simulink model "VVI"  (R2022b)
settings: Solver=FixedStepAuto  StartTime=0.0  StopTime=10.0  FixedStep=1e-3  RelTol=1e-3  EnableMultiTasking=on
undefined symbols (not defined in the file): D1, D10, D11, D12, D13, D2, D3, D4, D5, D7, D8, D9, PTA0, PTA1, PTA2, PTB23, PTB9, PTC17, PTC3, PTC4, PTD0, PTD1, PTD2, PTD3
libraries: frdmk64flib x12
settings Model: ExtModeTrigDuration=5  Creator=16475  LastModifiedBy=16475
settings OptimizationCC: EnhancedBackFolding=on  PassReuseOutputArgsAs=Individual arguments  ZeroExternalMemoryAtStartup=off  ZeroInternalMemoryAtStartup=off  MaxStackSize=64  OptimizeBlockOrder=speed  DifferentSizesBufferReuse=on  OptimizationCustomize=off  EfficientTunableParamExpr=on
settings DebuggingCC: ParameterTunabilityLossMsg=error
settings HardwareCC: ProdBitPerPointer=32  ProdBitPerSizeT=32  ProdBitPerPtrDiffT=32  ProdLargestAtomicInteger=Long  ProdLargestAtomicFloat=Double  ProdWordSize=32  ProdHWDeviceType=ARM Compatible->ARM Cortex
settings SFSimCC: MATLABDynamicMemAlloc=off
settings RTWCC: Description=Embedded Coder  SystemTargetFile=ert.tlc  HardwareBoard=NXP FRDM-K64F  TLCOptions="-aInlineSetEventsForThisBaseRateFcn=TLC_FALSE -aSuppressMultiTaskScheduler=TLC_FALSE  -aRateBasedStepFcn=0"  TemplateMakefile=ert_default_tmf  Toolchain=GNU Tools for ARM Embedded Processors
settings CodeAppCC: ForceParamTrailComments=on  IgnoreCustomStorageClasses=off  OperatorAnnotations=on  SimulinkDataObjDesc=on  SFDataObjDesc=on  InsertBlockDesc=on
settings ERTTargetCC: ExtModeTransport=4  ExtModeMexFile=sendToCommService

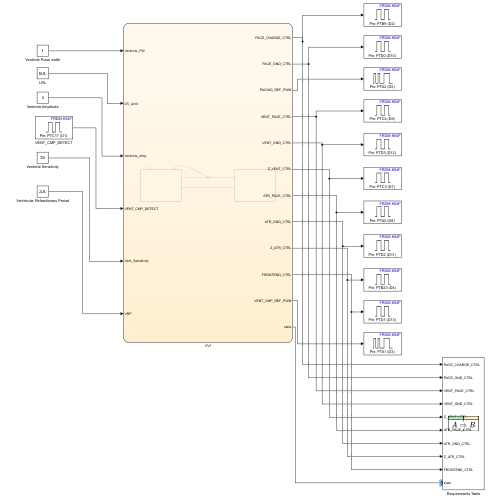
[thumbnail: Simulink's stored preview of the top-level diagram]
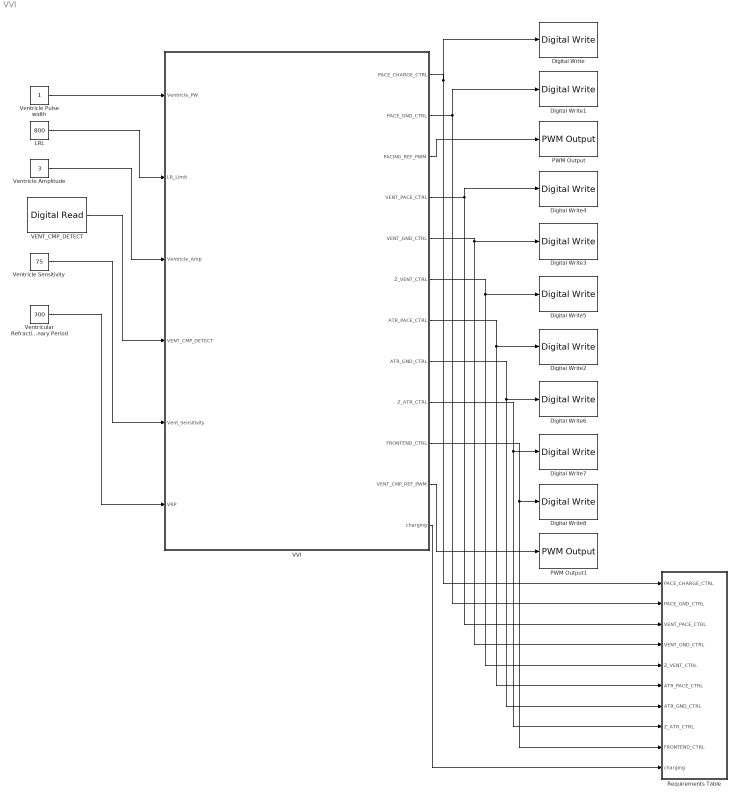
== system VVI ==
  Digital Write : frdmk64flib/Digital Write  Whichpin=PTB9 (D2)
  Digital Write1 : frdmk64flib/Digital Write  Whichpin=PTD0 (D10)
  Digital Write2 : frdmk64flib/Digital Write  Whichpin=PTA0 (D8)
  Digital Write3 : frdmk64flib/Digital Write  Whichpin=PTD3 (D12)
  Digital Write4 : frdmk64flib/Digital Write  Whichpin=PTC4 (D9)
  Digital Write5 : frdmk64flib/Digital Write  Whichpin=PTC3 (D7)
  Digital Write6 : frdmk64flib/Digital Write  Whichpin=PTD2 (D11)
  Digital Write7 : frdmk64flib/Digital Write  Whichpin=PTB23 (D4)
  Digital Write8 : frdmk64flib/Digital Write  Whichpin=PTD1 (D13)
  LRL : Constant  Value=800
  PWM Output : frdmk64flib/PWM Output  Whichpin=PTA2 (D5)  InitialFrequency=2000  InitialDutyCycle=0
  PWM Output1 : frdmk64flib/PWM Output  Whichpin=PTA1 (D3)  InitialFrequency=2000  InitialDutyCycle=0
  Requirements Table : Requirements Table  TreatAsAtomicUnit=on
  VENT_CMP_DETECT : frdmk64flib/Digital Read  Whichpin=PTC17 (D1)  SampleTime=-1
  VVI : Stateflow chart  TreatAsAtomicUnit=on
      settings: PortSchema="{\"entries\":[{\"content\":{\"sides\":[{\"content\":{\"connectorIds\":[\"In1\",\"In2\",\"In3\",\"In4\",\"In5\",\"In6\"]},\"type\":\"ConnectorPlacement.EquallySpacedRectSide\",\"uuid\":\"a3e94f58-3093-42a5-91db-f56c9d127bee\"},{\"content\":{\"connectorIds\":[\"Out1\",\"Out2\",\"Out3\",\"Out5\",\"Out4\",\"Out7\",\"Out6\",\"Out8\",\"Out9\",\"Out10\",\"Out11\",\"Out12\"],\"side\":\"RIGHT\"},\"type\":\"ConnectorPlacement.EquallySpacedRectSide\",\"uuid\":\"289ad049-9840-4721-af22-1385d5696f7c\"},{\"content\":{\"connectorIds\":[],\"side\":\"TOP\"},\"type\":\"ConnectorPlacement.EquallySpacedRectSide\",\"uuid\":\"4602f2ad-cb91-4c7a-9db6-6571445db01f\"}]},\"type\":\"ConnectorPlacement.EquallySpacedConnector\",\"uuid\":\"bfd50937-4990-4c1b-ba87-ff4dc7d3240f\"}],\"packageUris\":[\"http://schema.mathworks.com/mf0/Connector/R2020b\"],\"version\":\"1.0\"}"
  Ventricle Amplitude : Constant  Value=3
  Ventricle Pulse width : Constant
  Ventricle Sensitivity : Constant  Value=75
  Ventricular Refractionary Period : Constant  Value=300
  wires:
  LRL/1 -> VVI/2(LR_Limit)
  Ventricle Pulse width/1 -> VVI/1(Ventricle_PW)
  Ventricle Amplitude/1 -> VVI/3(Ventricle_Amp)
  VENT_CMP_DETECT/1 -> VVI/4(VENT_CMP_DETECT)
  VVI/11(VENT_CMP_REF_PWM) -> PWM Output1/1
  Ventricle Sensitivity/1 -> VVI/5(Vent_Sensitivity)
  Ventricular Refractionary Period/1 -> VVI/6(VRP)
  VVI/1(PACE_CHARGE_CTRL) -> Requirements Table/1(PACE_CHARGE_CTRL), Digital Write/1
  VVI/2(PACE_GND_CTRL) -> Requirements Table/2(PACE_GND_CTRL), Digital Write1/1
  VVI/3(PACING_REF_PWM) -> PWM Output/1
  VVI/5(VENT_PACE_CTRL) -> Requirements Table/3(VENT_PACE_CTRL), Digital Write4/1
  VVI/4(VENT_GND_CTRL) -> Requirements Table/4(VENT_GND_CTRL), Digital Write3/1
  VVI/7(Z_VENT_CTRL) -> Requirements Table/5(Z_VENT_CTRL), Digital Write5/1
  VVI/6(ATR_PACE_CTRL) -> Requirements Table/6(ATR_PACE_CTRL), Digital Write2/1
  VVI/8(ATR_GND_CTRL) -> Requirements Table/7(ATR_GND_CTRL), Digital Write6/1
  VVI/9(Z_ATR_CTRL) -> Requirements Table/8(Z_ATR_CTRL), Digital Write7/1
  VVI/10(FRONTEND_CTRL) -> Requirements Table/9(FRONTEND_CTRL), Digital Write8/1
  VVI/12(charging) -> Requirements Table/10(charging)

== stateflow chart VVI/VVI ==
  state Charging
    entry:
    ATR_PACE_CTRL = false;
    VENT_PACE_CTRL = false;
    PACING_REF_PWM = ((Ventricle_Amp/5)*100);
    PACE_CHARGE_CTRL = true;
    PACE_GND_CTRL = true;
    Z_ATR_CTRL = false;
    Z_VENT_CTRL = false;
    ATR_GND_CTRL = false;
    VENT_GND_CTRL = true;
    FRONTEND_CTRL = true;
    VENT_CMP_REF_PWM = Vent_Sensitivity;
    charging = true;
  state Discharging
    entry:
    PACE_CHARGE_CTRL = false;
    PACE_GND_CTRL = true;
    ATR_PACE_CTRL = false;
    VENT_PACE_CTRL = true;
    Z_ATR_CTRL = false;
    Z_VENT_CTRL = false;
    ATR_GND_CTRL = false;
    VENT_GND_CTRL = false;
    charging = false;
  (default) -> Charging
  (junction 36) -> Charging [order 2] : [VENT_CMP_DETECT == true]
  Charging -> (junction 36) : [after(VRP,msec)]
  (junction 36) -> Discharging [order 1] : [after(LR_Limit - VRP,msec)]
  Discharging -> Charging : [after(Ventricle_PW,msec)]
  data: Ventricle_PW input double; LR_Limit input double; PACE_CHARGE_CTRL output boolean; PACE_GND_CTRL output boolean; PACING_REF_PWM output double; VENT_GND_CTRL output boolean; VENT_PACE_CTRL output boolean; ATR_PACE_CTRL output boolean; Z_VENT_CTRL output boolean; Ventricle_Amp input double; ATR_GND_CTRL output boolean; Z_ATR_CTRL output boolean; VENT_CMP_DETECT input boolean; FRONTEND_CTRL output boolean; VENT_CMP_REF_PWM output double; Vent_Sensitivity input double; VRP input double; charging output

== stateflow chart VVI/Requirements Table ==
  (default) -> (junction 1073742466)
  (junction 1073742466) -> (junction 1073742467) : {
      | % SF_REQ_REV_07
      | }
  (junction 1073742467) -> (junction 1073742469) : {
      | % HEADER_ASSIGNMENTS
      |
      | }
  (junction 1073742469) -> (junction 1073742471) : {
      | % START_A_4
      | }
  (junction 1073742471) -> (junction 1073742473) : {
      | }
  (junction 1073742473) -> (junction 1073742475)
  (junction 1073742475) -> (junction 1073742477) : {
      | }
  (junction 1073742477) -> (junction 1073742479) : {
      | % END_A_4
      | }
  (junction 1073742479) -> (junction 1073742481) : {
      | % START_R_1
      | }
  (junction 1073742481) -> (junction 1073742483) : {
      | }
  (junction 1073742483) -> (junction 1073742485)
  (junction 1073742485) -> (junction 1073742487) [order 1] : [(((prev(charging)) == (prev(charging) == false)))]
  (junction 1073742485) -> (junction 1073742493) [order 2]
  (junction 1073742487) -> (junction 1073742489) : {
      | reqtable_postcondition((((PACE_CHARGE_CTRL) == (true))) && (((PACE_GND_CTRL) == (true))) && (((VENT_PACE_CTRL) == (false))) && (((VENT_GND_CTRL) == (true))) && (((Z_VENT_CTRL) == (false))) && (((ATR_PACE_CTRL) == (false))) && (((ATR_GND_CTRL) == (false))) && (((Z_ATR_CTRL) == (false))) && (((FRONTEND_CTRL) == (true))) && (((charging) == (true))), 'R:1');
      |
      |
      | }
  (junction 1073742489) -> (junction 1073742491) : {
      | }
  (junction 1073742491) -> (junction 1073742493)
  (junction 1073742493) -> (junction 1073742495)
  (junction 1073742495) -> (junction 1073742497) : {
      | % END_R_1
      | }
  (junction 1073742497) -> (junction 1073742499) : {
      | % START_R_7
      | }
  (junction 1073742499) -> (junction 1073742501) : {
      | }
  (junction 1073742501) -> (junction 1073742503)
  (junction 1073742503) -> (junction 1073742505) [order 1] : [(((prev(charging)) == (prev(charging) == true)))]
  (junction 1073742503) -> (junction 1073742511) [order 2]
  (junction 1073742505) -> (junction 1073742507) : {
      | reqtable_postcondition((((PACE_CHARGE_CTRL) == (false))) && (((PACE_GND_CTRL) == (true))) && (((VENT_PACE_CTRL) == (true))) && (((VENT_GND_CTRL) == (false))) && (((Z_VENT_CTRL) == (false))) && (((ATR_PACE_CTRL) == (false))) && (((ATR_GND_CTRL) == (false))) && (((Z_ATR_CTRL) == (false))) && (((FRONTEND_CTRL) == (false))) && (((charging) == (false))), 'R:2');
      |
      |
      | }
  (junction 1073742507) -> (junction 1073742509) : {
      | }
  (junction 1073742509) -> (junction 1073742511)
  (junction 1073742511) -> (junction 1073742513)
  (junction 1073742513) -> (junction 1073742515) : {
      | % END_R_7
      | }
  data: PACE_CHARGE_CTRL input boolean; PACE_GND_CTRL input boolean; VENT_PACE_CTRL input boolean; VENT_GND_CTRL input boolean; Z_VENT_CTRL input boolean; ATR_PACE_CTRL input boolean; ATR_GND_CTRL input boolean; Z_ATR_CTRL input boolean; FRONTEND_CTRL input boolean; charging input boolean
